simulink model "prescan_repl_getOutputs"  (R2019a)
settings: Solver=VariableStepAuto  StartTime=0.0  StopTime=100  RelTol=1e-3
libraries: ProSivic_Sensors x2, realtime_pacer_lib x1
settings Model: Creator=Markus Borg  LastModifiedBy=Markus Borg

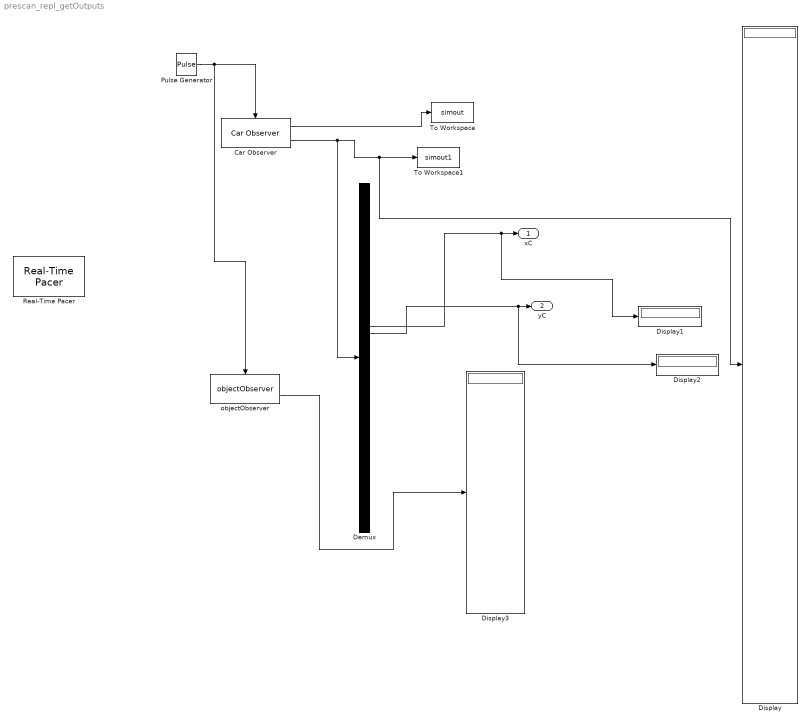
== system prescan_repl_getOutputs ==
  Car Observer : ProSivic_Sensors/Car Observer  SystemSampleTime=-1
      link override S-Function: topic=egocar_obs
  Demux : Demux  Outputs=40
  Display{,1..3} (4 alike) : Display
  Pulse Generator : DiscretePulseGenerator  PulseType=Time based  Period=0.5  PulseWidth=50
  Real-Time Pacer : realtime_pacer_lib/Real-Time Pacer  simTimePerRealTime=1
  To Workspace : ToWorkspace  VariableName=simout  SaveFormat=Timeseries  SampleTime=-1
  To Workspace1 : ToWorkspace  VariableName=simout1  SaveFormat=Timeseries  SampleTime=-1
  objectObserver : ProSivic_Sensors/objectObserver  topic=ped_obs
  xC : Outport
  yC : Outport  Port=2
  wires:
  Car Observer/2 -> Demux/1, Display/1, To Workspace1/1
  Pulse Generator/1 -> Car Observer/Trigger, objectObserver/Trigger
  Car Observer/1 -> To Workspace/1
  Demux/16 -> Display1/1, xC/1
  Demux/17 -> Display2/1, yC/1
  objectObserver/2 -> Display3/1
